simulink library "motohawk_control_primitives_lib"  (Simulink 7.5)
settings: Solver=ode45  SolverMode=SingleTasking  StartTime=0.0  StopTime=10.0  RelTol=1e-3
undefined symbols (not defined in the file): group, motohawk_vardec_config_group, motohawk_vardec_path, p, samp_time, SampleTime
libraries: MotoHawk_lib x103, motohawk_control_primitives_lib x29, simulink x11, AutoDoc_lib x4
(part 2 of 4)

== system motohawk_control_primitives_lib/Handoff Alpha ==
  note: Prevent divide by zero
  note: Convert a boolean input signal
      | to a more slowly ramping 'alpha' from 0 to 1
  in : Inport  OutDataType=sfix(16)  OutScaling=2^0
  up_tau : Inport  Port=2  OutDataType=sfix(16)  OutScaling=2^0
  down_tau : Inport  Port=3  OutDataType=sfix(16)  OutScaling=2^0
  Constant : Constant  Value=0  OutDataType=sfix(16)  OutScaling=2^0  OutDataTypeStr=Inherit: Inherit via back propagation
  Constant1 : Constant  OutDataType=sfix(16)  OutScaling=2^0  OutDataTypeStr=Inherit: Inherit via back propagation
  Multiport Switch : MultiPortSwitch  DataPortOrder=Zero-based contiguous  Inputs=2  zeroidx=on  SaturateOnIntegerOverflow=on  InputSameDT=on
  Product : Product  Inputs=*/  OutDataType=sfix(16)  OutScaling=2^0  SaturateOnIntegerOverflow=on  InputSameDT=on  OutDataTypeStr=Inherit: Same as first input
  Product1 : Product  Inputs=*/  OutDataType=sfix(16)  OutScaling=2^0  SaturateOnIntegerOverflow=on  InputSameDT=on  OutDataTypeStr=Inherit: Same as first input
  Ramp Down : Gain  Gain=-1  ParameterDataType=sfix(16)  ParameterScaling=2^0  OutDataType=sfix(16)  OutScaling=2^0  SaturateOnIntegerOverflow=on  OutDataTypeStr=Inherit: Same as input  ParamDataTypeStr=Inherit: Same as input
  Saturation : motohawk_control_primitives_lib/Saturation
  Signal Specification : SignalSpecification  DataType=boolean  OutDataType=sfix(16)  OutScaling=2^0  OutDataTypeStr=boolean
  Sum : Sum  Inputs=|++  OutDataType=sfix(16)  OutScaling=2^0  SaturateOnIntegerOverflow=on  InputSameDT=on
  Switch : Switch  Criteria=u2 > Threshold  SaturateOnIntegerOverflow=on  InputSameDT=on
  Switch1 : Switch  Criteria=u2 > Threshold  SaturateOnIntegerOverflow=on  InputSameDT=on
  motohawk_delta_time : MotoHawk_lib/Extra Development Blocks/motohawk_delta_time  samp_time=samp_time  init_val=0
  state : UnitDelay  SampleTime=-1
  alpha : Outport  OutDataType=sfix(16)  OutScaling=2^0
  wires:
  up_tau/1 -> Switch1/1, Switch1/2
  Switch1/1 -> Product1/2
  down_tau/1 -> Switch/1, Switch/2
  Switch/1 -> Product/2
  Signal Specification/1 -> Multiport Switch/1
  Ramp Down/1 -> Multiport Switch/2
  Saturation/1 -> alpha/1, state/1
  Constant1/1 -> Saturation/3
  Constant/1 -> Saturation/2
  state/1 -> Sum/2
  Sum/1 -> Saturation/1
  Multiport Switch/1 -> Sum/1
  Product1/1 -> Multiport Switch/3
  Product/1 -> Ramp Down/1
  in/1 -> Signal Specification/1
  motohawk_delta_time/1 -> Switch1/3, Product1/1, Switch/3, Product/1

== system motohawk_control_primitives_lib/Hysterisis ==
  HiThresh : Inport  OutDataType=sfix(16)  OutScaling=2^0
  LowThresh : Inport  Port=2  OutDataType=sfix(16)  OutScaling=2^0
  Signal : Inport  Port=3  OutDataType=sfix(16)  OutScaling=2^0
  Hysteresis : Subsystem
  LT : RelationalOperator  ZeroCross=off  InputSameDT=on
  LT1 : RelationalOperator  Operator=<=  ZeroCross=off  InputSameDT=on
  Logical Operator : Logic  Operator=NOT
  Switch2 : Switch  Threshold=1  ZeroCross=off  InputSameDT=on
  Threshold : Outport  OutDataType=sfix(16)  OutScaling=2^0
  wires:
  LT/1 -> Hysteresis/1(Hi)  "AboveHiTarget"
  LT1/1 -> Hysteresis/2(Lo)  "BelowLoTarget"
  Hysteresis/1("Out (Lo=0, Hi=1)") -> Logical Operator/1
  Logical Operator/1 -> Switch2/2
  HiThresh/1 -> Switch2/1, LT/2
  Switch2/1 -> Threshold/1
  LowThresh/1 -> Switch2/3, LT1/2
  Signal/1 -> LT/1, LT1/1

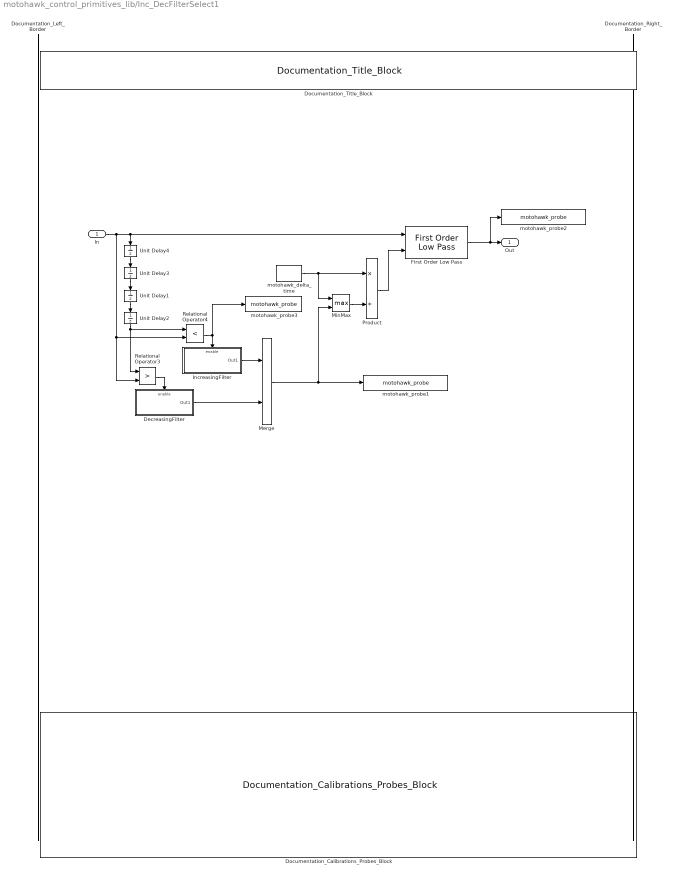
== system motohawk_control_primitives_lib/Inc_DecFilterSelect1 ==
  In : Inport  OutDataType=sfix(16)  OutScaling=2^0
  DecreasingFilter : Subsystem  TreatAsAtomicUnit=on
  Documentation_Calibrations_Probes_Block : AutoDoc_lib/Documentation_Calibrations_Probes_Block
  Documentation_Left_Border : AutoDoc_lib/Documentation_Left_Border  layout=Portrait
  Documentation_Right_Border : AutoDoc_lib/Documentation_Right_Border  layout=Portrait
  Documentation_Title_Block : AutoDoc_lib/Documentation_Title_Block
  First Order Low Pass : motohawk_control_primitives_lib/First Order Low Pass
  IncreasingFilter : Subsystem  TreatAsAtomicUnit=on
  Merge : Merge
  MinMax : MinMax  Function=max  Inputs=2  OutDataType=sfix(16)  OutScaling=2^0  SaturateOnIntegerOverflow=on  InputSameDT=on
  Product : Product  Inputs=*/  OutDataType=sfix(16)  OutScaling=2^0  SaturateOnIntegerOverflow=on  InputSameDT=on  OutDataTypeStr=Inherit: Same as first input
  Relational Operator3 : RelationalOperator  Operator=>  LogicOutDataTypeMode=boolean  OutDataTypeStr=boolean
  Relational Operator4 : RelationalOperator  Operator=<  LogicOutDataTypeMode=boolean  OutDataTypeStr=boolean
  Unit Delay{1..4} (4 alike) : UnitDelay  SampleTime=-1
  motohawk_delta_time : MotoHawk_lib/Extra Development Blocks/motohawk_delta_time  samp_time=.005  init_val=.005
  motohawk_probe1 : MotoHawk_lib/Calibration & Probing Blocks/motohawk_probe  nam=[nam 'FilterConst']  show_more=on  name_source=Use Parameter  read_level=1  view_as=Number  enum_struct={'Disabled', 'Enabled'}  vector_style=Wide Row  use_help_units=off  help=''  units=''  use_header_enum=off  row_header_enum={}  col_header_enum={}  use_precision=off  precision=''  gain=1  offset=0  exp=1  use_mototune_group=on  mototune_group=grp_dis
  motohawk_probe2 : MotoHawk_lib/Calibration & Probing Blocks/motohawk_probe  nam=[nam 'Filtered']  show_more=on  name_source=Use Parameter  read_level=1  view_as=Number  enum_struct={'Disabled', 'Enabled'}  vector_style=Wide Row  use_help_units=off  help=''  units=''  use_header_enum=off  row_header_enum={}  col_header_enum={}  use_precision=off  precision=''  gain=1  offset=0  exp=1  use_mototune_group=on  mototune_group=grp_dis
  motohawk_probe3 : MotoHawk_lib/Calibration & Probing Blocks/motohawk_probe  nam=[nam 'Direction']  show_more=on  name_source=Use Parameter  read_level=1  view_as=Enumeration  enum_struct={'Decreasing', 'Increasing'}  vector_style=Wide Row  use_help_units=on  help=''  units=''  use_header_enum=off  row_header_enum={}  col_header_enum={}  use_precision=off  precision=''  gain=1  offset=0  exp=1  use_mototune_group=on  mototune_group=grp_dis
  Out : Outport  OutDataType=sfix(16)  OutScaling=2^0
  wires:
  Unit Delay4/1 -> Unit Delay3/1
  Unit Delay3/1 -> Unit Delay1/1
  Unit Delay1/1 -> Unit Delay2/1
  Unit Delay2/1 -> Relational Operator4/1, Relational Operator3/1
  Product/1 -> First Order Low Pass/2
  First Order Low Pass/1 -> Out/1, motohawk_probe2/1
  motohawk_delta_time/1 -> MinMax/1, Product/1
  MinMax/1 -> Product/2
  Merge/1 -> MinMax/2, motohawk_probe1/1
  Relational Operator4/1 -> motohawk_probe3/1, IncreasingFilter/Enable
  Relational Operator3/1 -> DecreasingFilter/Enable
  DecreasingFilter/1(Out1) -> Merge/2
  IncreasingFilter/1(Out1) -> Merge/1
  In/1 -> First Order Low Pass/1, Unit Delay4/1, Relational Operator3/2, Relational Operator4/2

== system motohawk_control_primitives_lib/Integrator ==
  note: Discrete Integrator,
      | with output and state saturation.
  In : Inport  OutDataType=sfix(16)  OutScaling=2^0
  Rst : Inport  Port=2  OutDataType=sfix(16)  OutScaling=2^0
  IC : Inport  Port=3  OutDataType=sfix(16)  OutScaling=2^0
  Min : Inport  Port=4  OutDataType=sfix(16)  OutScaling=2^0
  Max : Inport  Port=5  OutDataType=sfix(16)  OutScaling=2^0
  Data Type Conversion : DataTypeConversion  OutDataTypeMode=boolean  OutDataType=sfix(16)  OutScaling=2^0  OutDataTypeStr=boolean  RndMeth=Zero
  Product : Product  OutDataType=sfix(16)  OutScaling=2^0  SaturateOnIntegerOverflow=on  InputSameDT=on  OutDataTypeStr=Inherit: Same as first input
  Saturation : motohawk_control_primitives_lib/Saturation
  Sum : Sum  Inputs=++|  OutDataType=sfix(16)  OutScaling=2^0  SaturateOnIntegerOverflow=on  InputSameDT=on
  Switch1 : Switch  Threshold=1  ZeroCross=off  SaturateOnIntegerOverflow=on  InputSameDT=on
  Unit Delay : UnitDelay  SampleTime=-1
  motohawk_delta_time : MotoHawk_lib/Extra Development Blocks/motohawk_delta_time  samp_time=-1  init_val=0
  Out : Outport  OutDataType=sfix(16)  OutScaling=2^0
  wires:
  Saturation/1 -> Unit Delay/1
  Sum/1 -> Saturation/1
  Switch1/1 -> Out/1, Sum/1
  motohawk_delta_time/1 -> Product/2
  In/1 -> Product/1
  Product/1 -> Sum/2
  Unit Delay/1 -> Switch1/3
  Rst/1 -> Data Type Conversion/1
  Data Type Conversion/1 -> Switch1/2
  Min/1 -> Saturation/2
  Max/1 -> Saturation/3
  IC/1 -> Switch1/1

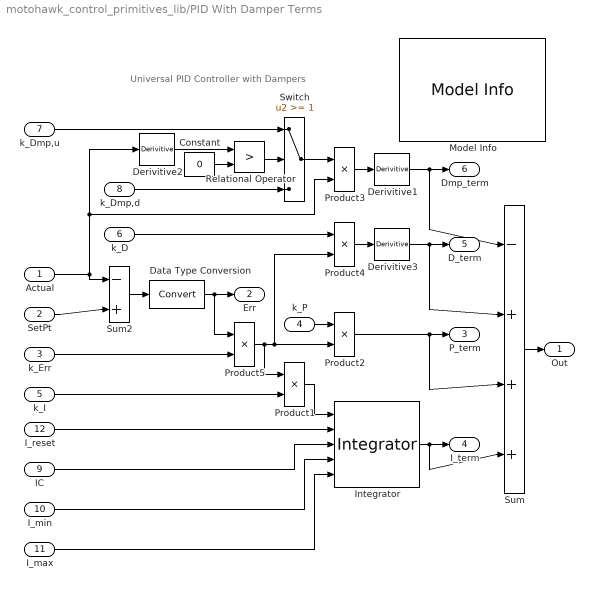
== system motohawk_control_primitives_lib/PID With Damper Terms ==
  note: Universal PID Controller
      | with Dampers
  Actual : Inport  OutDataType=sfix(16)  OutScaling=2^0
  SetPt : Inport  Port=2  OutDataType=sfix(16)  OutScaling=2^0
  k_Err : Inport  Port=3  OutDataType=sfix(16)  OutScaling=2^0
  k_P : Inport  Port=4  OutDataType=sfix(16)  OutScaling=2^0
  k_I : Inport  Port=5  OutDataType=sfix(16)  OutScaling=2^0
  k_D : Inport  Port=6  OutDataType=sfix(16)  OutScaling=2^0
  k_Dmp,u : Inport  Port=7  OutDataType=sfix(16)  OutScaling=2^0
  k_Dmp,d : Inport  Port=8  OutDataType=sfix(16)  OutScaling=2^0
  IC : Inport  Port=9  OutDataType=sfix(16)  OutScaling=2^0
  I_min : Inport  Port=10  OutDataType=sfix(16)  OutScaling=2^0
  I_max : Inport  Port=11  OutDataType=sfix(16)  OutScaling=2^0
  I_reset : Inport  Port=12  OutDataType=sfix(16)  OutScaling=2^0
  Constant : Constant  Value=0  OutDataType=sfix(16)  OutScaling=2^0  OutDataTypeStr=Inherit: Inherit via back propagation
  Data Type Conversion : DataTypeConversion  OutDataType=sfix(16)  OutScaling=2^0  SaturateOnIntegerOverflow=on  RndMeth=Zero
  Derivitive1 : motohawk_control_primitives_lib/Derivitive  samp_time=samp_time
  Derivitive2 : motohawk_control_primitives_lib/Derivitive  samp_time=samp_time
  Derivitive3 : motohawk_control_primitives_lib/Derivitive  samp_time=samp_time
  Integrator : motohawk_control_primitives_lib/Integrator  samp_time=samp_time
  Model Info : simulink/Model-Wide Utilities/Model Info  InitialBlockCM=None  BlockCM=None  Frame=on  DisplayStringWithTags=|  HorizontalTextAlignment=Center  LeftAlignmentValue=0.5  SourceBlockDiagram=motohawk_control_primitives_lib  TagMaxNumber=20
      | Model Info:
      | Author: Suhre, Poorman
      | %<Created>
      | %<ModifiedDate>
      | Version: %<ModelVersion>
      | MotoTron Confidential
      | and Propietary
  Product{1..5} (5 alike) : Product  OutDataType=sfix(16)  OutScaling=2^0  InputSameDT=on  OutDataTypeStr=Inherit: Same as first input
  Relational Operator : RelationalOperator  Operator=>  ZeroCross=off  InputSameDT=on
  Sum : Sum  Inputs=-|+|+|+  OutDataType=sfix(16)  OutScaling=2^0  SaturateOnIntegerOverflow=on  InputSameDT=on  OutDataTypeStr=Inherit: Same as first input
  Sum2 : Sum  Inputs=-|+  OutDataType=sfix(16)  OutScaling=2^0  SaturateOnIntegerOverflow=on  InputSameDT=on  OutDataTypeStr=Inherit: Same as first input
  Switch : Switch  Threshold=1  ZeroCross=off  InputSameDT=on
  Out : Outport  OutDataType=sfix(16)  OutScaling=2^0
  Err : Outport  Port=2  OutDataType=sfix(16)  OutScaling=2^0
  P_term : Outport  Port=3  OutDataType=sfix(16)  OutScaling=2^0
  I_term : Outport  Port=4  OutDataType=sfix(16)  OutScaling=2^0
  D_term : Outport  Port=5  OutDataType=sfix(16)  OutScaling=2^0
  Dmp_term : Outport  Port=6  OutDataType=sfix(16)  OutScaling=2^0
  wires:
  Product3/1 -> Derivitive1/1
  k_Dmp,u/1 -> Switch/1
  k_Dmp,d/1 -> Switch/3
  Switch/1 -> Product3/1
  Derivitive2/1 -> Relational Operator/1
  Relational Operator/1 -> Switch/2
  Constant/1 -> Relational Operator/2
  I_max/1 -> Integrator/5
  I_min/1 -> Integrator/4
  Data Type Conversion/1 -> Product5/1, Err/1
  k_Err/1 -> Product5/2
  I_reset/1 -> Integrator/2
  Actual/1 -> Sum2/1, Derivitive2/1, Product3/2
  k_P/1 -> Product2/1
  k_I/1 -> Product1/2
  Product1/1 -> Integrator/1
  Product2/1 -> P_term/1, Sum/3
  Integrator/1 -> I_term/1, Sum/4
  Sum/1 -> Out/1
  IC/1 -> Integrator/3
  Product5/1 -> Product1/1, Product2/2, Product4/2
  Sum2/1 -> Data Type Conversion/1
  SetPt/1 -> Sum2/2
  k_D/1 -> Product4/1
  Product4/1 -> Derivitive3/1
  Derivitive3/1 -> D_term/1, Sum/2
  Derivitive1/1 -> Dmp_term/1, Sum/1

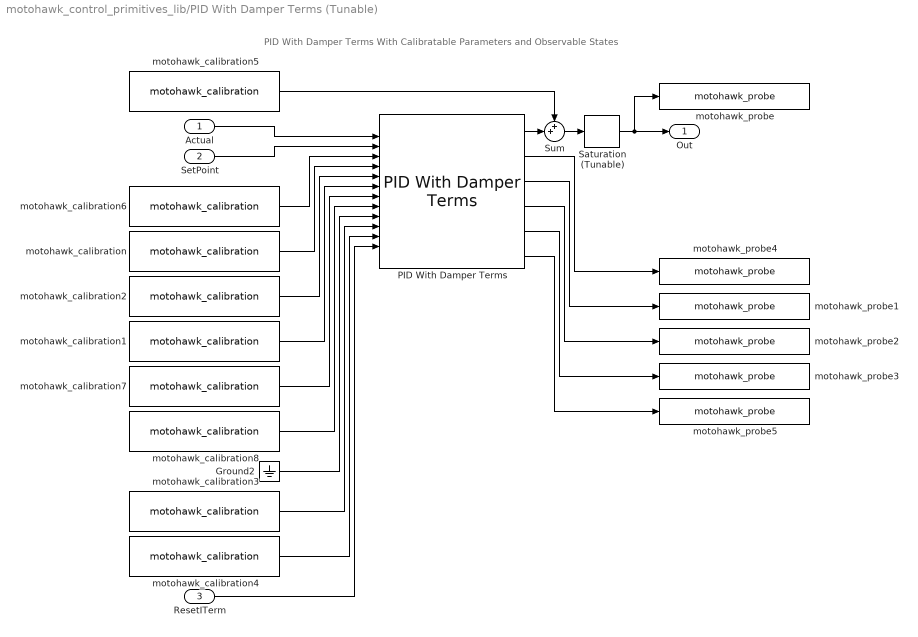
== system motohawk_control_primitives_lib/PID With Damper Terms (Tunable) ==
  note: PID With Damper Terms
      | With Calibratable Parameters and Observable States
  Actual : Inport  OutDataType=sfix(16)  OutScaling=2^0
  SetPoint : Inport  Port=2  OutDataType=sfix(16)  OutScaling=2^0
  ResetITerm : Inport  Port=3  OutDataType=sfix(16)  OutScaling=2^0
  Ground2 : Ground
  PID With Damper Terms : motohawk_control_primitives_lib/PID With Damper Terms  Description=|  samp_time=SampleTime
      | /* Name: ErrorGain Unit:mult ClassID:VAR StorageID:FLASH Access:RW4+RW3+NA2+NA1 TypeID:UINT4                   
      |    Gain:0.000000001 Min:0.000000000 Max:4.000000000 Format:10.9 UpdateID:REMOTE Help:"This gain is applied to "
      |    "the error term before it is used to calculate the P, I and D terms." VardecSig:6C */                       
      |                                                                                                                
      | /* Name: ITermLowerLim Unit:0 ClassID:VAR StorageID:FLASH Access:RW4+RW3+NA2+NA1 TypeID:SINT2 Gain:0.1         
      |    Min:-3276.8 Max:3276.7 Format:5.1 UpdateID:REMOTE Help:"Lower limit on the I-term value." VardecSig:6C */   
      |                                                                                                                
      | /* Name: ITermUpperLim ClassID:VAR StorageID:FLASH Access:RW4+RW3+NA2+NA1 TypeID:SINT2 Gain:0.1 Min:-3276.8    
      |    Max:3276.7 Format:5.1 UpdateID:REMOTE Help:"Upper limit on I-term value." VardecSig:6C */                   
      |                                                                                                                
      | /* Name: PIDOutLowerLim ClassID:VAR StorageID:FLASH Access:RW4+RW3+NA2+NA1 TypeID:SINT2 Gain:0.1               
      |    Min:-3276.8 Max:3276.7 Format:5.1 UpdateID:REMOTE Help:"Lower limit on PID output." VardecSig:6C */         
      |                                                                                                                
      | /* Name: PIDOutUpperLim ClassID:VAR StorageID:FLASH Access:RW4+RW3+NA2+NA1 TypeID:SINT2 Gain:0.1               
      |    Min:-3276.8 Max:3276.7 Format:3.1 UpdateID:REMOTE Help:"Upper limit on PID output." VardecSig:6C */         
      |                                                                                                                
      | /* Name: PIDError ClassID:VAR StorageID:RAM Access:RO4+RO3+NA2+NA1 TypeID:SINT2 Gain:1 Min:-32768.00           
      |    Max:32767.00 Format:4.2 UpdateID:BACKGND Help:"Current controller error input value." VardecSig:6C */       
      |                                                                                                                
      | /* Name: PTerm ClassID:VAR StorageID:RAM Access:RO4+RO3+NA2+NA1 TypeID:SINT2 Gain:1 Min:-32768.00              
      |    Max:32767.00 Format:4.2 UpdateID:BACKGND Help:"Current P-term value" VardecSig:6C */                        
      |                                                                                                                
      | /* Name: ITerm ClassID:VAR StorageID:RAM Access:RO4+RO3+NA2+NA1 TypeID:SINT2 Gain:1 Min:-32768.00              
      |    Max:32767.00 Format:4.2 UpdateID:BACKGND Help:"Current I-term value" VardecSig:6C */                        
      |                                                                                                                
      | /* Name: DTerm ClassID:VAR StorageID:RAM Access:RO4+RO3+NA2+NA1 TypeID:SINT2 Gain:1 Min:-32768.00              
      |    Max:32767.00 Format:4.2 UpdateID:BACKGND Help:"Current D-term value" VardecSig:6C */                        
      |                                                                                                                
      | /* Name: DamperTerm ClassID:VAR StorageID:RAM Access:RO4+RO3+NA2+NA1 TypeID:SINT2 Gain:1 Min:-32768.00         
      |    Max:32767.00 Format:4.2 UpdateID:BACKGND Help:"Current Damper-term value" VardecSig:6C */                   
      |                                                                                                                
      | /* Name: PIDOutput ClassID:VAR StorageID:FLASH Access:RW4+RW3+NA2+NA1 TypeID:SINT2 Gain:1 Min:-32768.00        
      |    Max:32767.00 Format:4.2 UpdateID:REMOTE Help:"PID current output." VardecSig:6C */
  Saturation (Tunable) : motohawk_control_primitives_lib/Saturation (Tunable)  prefix=prefix  units=units  grp=grp
  Sum : Sum  Inputs=++|  OutDataType=sfix(16)  OutScaling=2^0  InputSameDT=on
  motohawk_calibration : MotoHawk_lib/Calibration & Probing Blocks/motohawk_calibration  nam=[prefix 'PGain']  val=1  storage=Calibration  show_more=on  name_source=Use Parameter  data_type=Inherit from 'Default Value'  read_level=1  write_level=1  ovr_cals=on  view_as=Number  enum_struct={'Disabled', 'Enabled'}  vector_style=Wide Row  use_help_units=on  help='PID Proportional Gain'  units='mult'  use_header_enum=off  row_header_enum={}  col_header_enum={}  use_min_max=off  min_val=-inf  max_val=inf  use_precision=off  precision=''  gain=1  offset=0  exp=1  use_mototune_group=on  mototune_group=grp
  motohawk_calibration1 : MotoHawk_lib/Calibration & Probing Blocks/motohawk_calibration  nam=[prefix 'DGain']  val=1  storage=Calibration  show_more=on  name_source=Use Parameter  data_type=Inherit from 'Default Value'  read_level=1  write_level=1  ovr_cals=on  view_as=Number  enum_struct={'Disabled', 'Enabled'}  vector_style=Wide Row  use_help_units=on  help='PID Derivative Gain'  units='mult'  use_header_enum=off  row_header_enum={}  col_header_enum={}  use_min_max=off  min_val=-inf  max_val=inf  use_precision=off  precision=''  gain=1  offset=0  exp=1  use_mototune_group=on  mototune_group=grp
  motohawk_calibration2 : MotoHawk_lib/Calibration & Probing Blocks/motohawk_calibration  nam=[prefix 'IGain']  val=1  storage=Calibration  show_more=on  name_source=Use Parameter  data_type=Inherit from 'Default Value'  read_level=1  write_level=1  ovr_cals=on  view_as=Number  enum_struct={'Disabled', 'Enabled'}  vector_style=Wide Row  use_help_units=on  help='PID Integral Gain'  units='mult'  use_header_enum=off  row_header_enum={}  col_header_enum={}  use_min_max=off  min_val=-inf  max_val=inf  use_precision=off  precision=''  gain=1  offset=0  exp=1  use_mototune_group=on  mototune_group=grp
  motohawk_calibration3 : MotoHawk_lib/Calibration & Probing Blocks/motohawk_calibration  nam=[prefix 'IMin']  val=0  storage=Calibration  show_more=on  name_source=Use Parameter  data_type=Inherit from 'Default Value'  read_level=1  write_level=1  ovr_cals=on  view_as=Number  enum_struct={'Disabled', 'Enabled'}  vector_style=Wide Row  use_help_units=on  help='PID Integrator Lower Limit'  units=units  use_header_enum=off  row_header_enum={}  col_header_enum={}  use_min_max=off  min_val=-inf  max_val=inf  use_precision=off  precision=''  gain=1  offset=0  exp=1  use_mototune_group=on  mototune_group=grp
  motohawk_calibration4 : MotoHawk_lib/Calibration & Probing Blocks/motohawk_calibration  nam=[prefix 'IMax']  val=1  storage=Calibration  show_more=on  name_source=Use Parameter  data_type=Inherit from 'Default Value'  read_level=1  write_level=1  ovr_cals=on  view_as=Number  enum_struct={'Disabled', 'Enabled'}  vector_style=Wide Row  use_help_units=on  help='PID Integrator Upper Limit'  units=units  use_header_enum=off  row_header_enum={}  col_header_enum={}  use_min_max=off  min_val=-inf  max_val=inf  use_precision=off  precision=''  gain=1  offset=0  exp=1  use_mototune_group=on  mototune_group=grp
  motohawk_calibration5 : MotoHawk_lib/Calibration & Probing Blocks/motohawk_calibration  nam=[prefix 'DCOffset']  val=0  storage=Calibration  show_more=on  name_source=Use Parameter  data_type=Inherit from 'Default Value'  read_level=1  write_level=1  ovr_cals=on  view_as=Number  enum_struct={'Disabled', 'Enabled'}  vector_style=Wide Row  use_help_units=on  help='PID Output DC Offset'  units=units  use_header_enum=off  row_header_enum={}  col_header_enum={}  use_min_max=off  min_val=-inf  max_val=inf  use_precision=off  precision=''  gain=1  offset=0  exp=1  use_mototune_group=on  mototune_group=grp
  motohawk_calibration6 : MotoHawk_lib/Calibration & Probing Blocks/motohawk_calibration  nam=[prefix 'ErrorGain']  val=1  storage=Calibration  show_more=on  name_source=Use Parameter  data_type=Inherit from 'Default Value'  read_level=1  write_level=1  ovr_cals=on  view_as=Number  enum_struct={'Disabled', 'Enabled'}  vector_style=Wide Row  use_help_units=on  help='PID Error Gain'  units='mult'  use_header_enum=off  row_header_enum={}  col_header_enum={}  use_min_max=off  min_val=-inf  max_val=inf  use_precision=off  precision=''  gain=1  offset=0  exp=1  use_mototune_group=on  mototune_group=grp
  motohawk_calibration7 : MotoHawk_lib/Calibration & Probing Blocks/motohawk_calibration  nam=[prefix 'DampGainUp']  val=1  storage=Calibration  show_more=on  name_source=Use Parameter  data_type=Inherit from 'Default Value'  read_level=1  write_level=1  ovr_cals=on  view_as=Number  enum_struct={'Disabled', 'Enabled'}  vector_style=Wide Row  use_help_units=on  help='PID Damper Gain - Up Direction'  units='mult'  use_header_enum=off  row_header_enum={}  col_header_enum={}  use_min_max=off  min_val=-inf  max_val=inf  use_precision=off  precision=''  gain=1  offset=0  exp=1  use_mototune_group=on  mototune_group=grp
  motohawk_calibration8 : MotoHawk_lib/Calibration & Probing Blocks/motohawk_calibration  nam=[prefix 'DampGainDown']  val=1  storage=Calibration  show_more=on  name_source=Use Parameter  data_type=Inherit from 'Default Value'  read_level=1  write_level=1  ovr_cals=on  view_as=Number  enum_struct={'Disabled', 'Enabled'}  vector_style=Wide Row  use_help_units=on  help='PID Damper Gain - Down Direction'  units='mult'  use_header_enum=off  row_header_enum={}  col_header_enum={}  use_min_max=off  min_val=-inf  max_val=inf  use_precision=off  precision=''  gain=1  offset=0  exp=1  use_mototune_group=on  mototune_group=grp
  motohawk_probe : MotoHawk_lib/Calibration & Probing Blocks/motohawk_probe  nam=[prefix 'Out']  show_more=on  name_source=Use Parameter  read_level=1  view_as=Number  enum_struct={'Disabled', 'Enabled'}  vector_style=Wide Row  use_help_units=on  help='PID Final Output'  units=units  use_header_enum=off  row_header_enum={}  col_header_enum={}  use_precision=off  precision=''  gain=1  offset=0  exp=1  use_mototune_group=on  mototune_group=grp
  motohawk_probe1 : MotoHawk_lib/Calibration & Probing Blocks/motohawk_probe  nam=[prefix 'PTerm']  show_more=on  name_source=Use Parameter  read_level=1  view_as=Number  enum_struct={'Disabled', 'Enabled'}  vector_style=Wide Row  use_help_units=on  help='PID Proportional Term'  units=units  use_header_enum=off  row_header_enum={}  col_header_enum={}  use_precision=off  precision=''  gain=1  offset=0  exp=1  use_mototune_group=on  mototune_group=grp
  motohawk_probe2 : MotoHawk_lib/Calibration & Probing Blocks/motohawk_probe  nam=[prefix 'ITerm']  show_more=on  name_source=Use Parameter  read_level=1  view_as=Number  enum_struct={'Disabled', 'Enabled'}  vector_style=Wide Row  use_help_units=on  help='PID Integrator Term'  units=units  use_header_enum=off  row_header_enum={}  col_header_enum={}  use_precision=off  precision=''  gain=1  offset=0  exp=1  use_mototune_group=on  mototune_group=grp
  motohawk_probe3 : MotoHawk_lib/Calibration & Probing Blocks/motohawk_probe  nam=[prefix 'DTerm']  show_more=on  name_source=Use Parameter  read_level=1  view_as=Number  enum_struct={'Disabled', 'Enabled'}  vector_style=Wide Row  use_help_units=on  help='PID Derivative Term'  units=units  use_header_enum=off  row_header_enum={}  col_header_enum={}  use_precision=off  precision=''  gain=1  offset=0  exp=1  use_mototune_group=on  mototune_group=grp
  motohawk_probe4 : MotoHawk_lib/Calibration & Probing Blocks/motohawk_probe  nam=[prefix 'Error']  show_more=on  name_source=Use Parameter  read_level=1  view_as=Number  enum_struct={'Disabled', 'Enabled'}  vector_style=Wide Row  use_help_units=on  help='PID Error Term'  units=units  use_header_enum=off  row_header_enum={}  col_header_enum={}  use_precision=off  precision=''  gain=1  offset=0  exp=1  use_mototune_group=on  mototune_group=grp
  motohawk_probe5 : MotoHawk_lib/Calibration & Probing Blocks/motohawk_probe  nam=[prefix 'DampTerm']  show_more=on  name_source=Use Parameter  read_level=1  view_as=Number  enum_struct={'Disabled', 'Enabled'}  vector_style=Wide Row  use_help_units=on  help='PID Damper Term'  units=units  use_header_enum=off  row_header_enum={}  col_header_enum={}  use_precision=off  precision=''  gain=1  offset=0  exp=1  use_mototune_group=on  mototune_group=grp
  Out : Outport  OutDataType=sfix(16)  OutScaling=2^0
  wires:
  motohawk_calibration5/1 -> Sum/1
  Sum/1 -> Saturation (Tunable)/1
  ResetITerm/1 -> PID With Damper Terms/12
  Ground2/1 -> PID With Damper Terms/9
  motohawk_calibration1/1 -> PID With Damper Terms/6
  motohawk_calibration2/1 -> PID With Damper Terms/5
  motohawk_calibration/1 -> PID With Damper Terms/4
  PID With Damper Terms/3 -> motohawk_probe1/1
  Actual/1 -> PID With Damper Terms/1
  SetPoint/1 -> PID With Damper Terms/2
  PID With Damper Terms/1 -> Sum/2
  motohawk_calibration6/1 -> PID With Damper Terms/3
  motohawk_calibration3/1 -> PID With Damper Terms/10
  motohawk_calibration4/1 -> PID With Damper Terms/11
  PID With Damper Terms/4 -> motohawk_probe2/1
  PID With Damper Terms/5 -> motohawk_probe3/1
  PID With Damper Terms/2 -> motohawk_probe4/1
  motohawk_calibration7/1 -> PID With Damper Terms/7
  motohawk_calibration8/1 -> PID With Damper Terms/8
  PID With Damper Terms/6 -> motohawk_probe5/1
  Saturation (Tunable)/1 -> Out/1, motohawk_probe/1

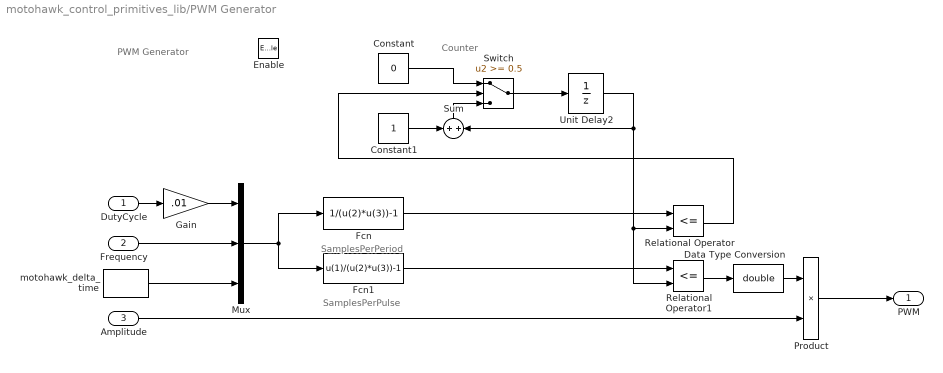
== system motohawk_control_primitives_lib/PWM Generator ==
  note: Counter
  note: PWM Generator
  note: SamplesPerPulse
  note: SamplesPerPeriod
  DutyCycle : Inport  OutDataType=sfix(16)  OutScaling=2^0
  Frequency : Inport  Port=2  OutDataType=sfix(16)  OutScaling=2^0
  Amplitude : Inport  Port=3  OutDataType=sfix(16)  OutScaling=2^0
  Enable : EnablePort  StatesWhenEnabling=reset
  Constant : Constant  Value=0  OutDataType=sfix(16)  OutScaling=2^0
  Constant1 : Constant  OutDataType=sfix(16)  OutScaling=2^0
  Data Type Conversion : DataTypeConversion  OutDataTypeMode=double  OutDataType=sfix(16)  OutScaling=2^0  OutDataTypeStr=double  SaturateOnIntegerOverflow=on  RndMeth=Zero
  Fcn : Fcn  Expr=1/(u(2)*u(3))-1
  Fcn1 : Fcn  Expr=u(1)/(u(2)*u(3))-1
  Gain : Gain  Gain=.01  ParameterDataType=sfix(16)  ParameterScaling=2^0  OutDataType=sfix(16)  OutScaling=2^0  SaturateOnIntegerOverflow=on  OutDataTypeStr=Inherit: Same as input  ParamDataTypeStr=Inherit: Same as input
  Mux : Mux  Inputs=3
  Product : Product  OutDataType=sfix(16)  OutScaling=2^0  SaturateOnIntegerOverflow=on  OutDataTypeStr=Inherit: Same as first input
  Relational Operator : RelationalOperator  Operator=<=
  Relational Operator1 : RelationalOperator  Operator=<=
  Sum : Sum  OutDataType=sfix(16)  OutScaling=2^0  SaturateOnIntegerOverflow=on  InputSameDT=on  OutDataTypeStr=Inherit: Same as first input
  Switch : Switch  Threshold=0.5  SaturateOnIntegerOverflow=on  InputSameDT=on
  Unit Delay2 : UnitDelay  SampleTime=-1
  motohawk_delta_time : MotoHawk_lib/Extra Development Blocks/motohawk_delta_time  samp_time=-1  init_val=.005
  PWM : Outport  OutDataType=sfix(16)  OutScaling=2^0  OutputWhenDisabled=reset  InitialOutput=0
  wires:
  Relational Operator/1 -> Switch/2
  Constant1/1 -> Sum/1
  Gain/1 -> Mux/1
  Data Type Conversion/1 -> Product/1
  Unit Delay2/1 -> Relational Operator1/2, Relational Operator/2, Sum/2
  Switch/1 -> Unit Delay2/1
  Constant/1 -> Switch/1
  Sum/1 -> Switch/3
  Amplitude/1 -> Product/2
  Product/1 -> PWM/1
  Relational Operator1/1 -> Data Type Conversion/1
  Fcn1/1 -> Relational Operator1/1
  Fcn/1 -> Relational Operator/1
  Mux/1 -> Fcn1/1, Fcn/1
  motohawk_delta_time/1 -> Mux/3
  Frequency/1 -> Mux/2
  DutyCycle/1 -> Gain/1

== system motohawk_control_primitives_lib/Per Cylinder Tables ==
  y_Idx : Inport  OutDataType=sfix(16)  OutScaling=2^0
  X_Idx : Inport  Port=2  OutDataType=sfix(16)  OutScaling=2^0
  Cyl : Inport  Port=3  OutDataType=sfix(16)  OutScaling=2^0
  Cyl1 : Subsystem  TreatAsAtomicUnit=on
  Cyl2 : Subsystem  TreatAsAtomicUnit=on
  Cyl3 : Subsystem  TreatAsAtomicUnit=on
  Cyl4 : Subsystem  TreatAsAtomicUnit=on
  Cyl5 : Subsystem  TreatAsAtomicUnit=on
  Cyl6 : Subsystem  TreatAsAtomicUnit=on
  Data Type Conversion : DataTypeConversion  OutDataTypeMode=uint8  OutDataType=sfix(16)  OutScaling=2^0  OutDataTypeStr=uint8  SaturateOnIntegerOverflow=on  RndMeth=Zero
  Multiport Switch : MultiPortSwitch  Inputs=6  zeroidx=off  SaturateOnIntegerOverflow=on
  Switch Case : SwitchCase  CaseConditions={1,2,3,4,5,6}  ShowDefaultCase=off
  Out1 : Outport  OutDataType=sfix(16)  OutScaling=2^0
  wires:
  Multiport Switch/1 -> Out1/1
  Cyl6/1(Value) -> Multiport Switch/7
  Cyl5/1(Value) -> Multiport Switch/6
  Cyl4/1(Value) -> Multiport Switch/5
  Cyl3/1(Value) -> Multiport Switch/4
  Cyl2/1(Value) -> Multiport Switch/3
  Cyl1/1(Value) -> Multiport Switch/2
  Data Type Conversion/1 -> Multiport Switch/1, Switch Case/1
  Switch Case/6 -> Cyl6/Action
  Switch Case/5 -> Cyl5/Action
  Switch Case/4 -> Cyl4/Action
  Switch Case/3 -> Cyl3/Action
  Switch Case/2 -> Cyl2/Action
  Switch Case/1 -> Cyl1/Action
  y_Idx/1 -> Cyl6/1(Row), Cyl5/1(Row), Cyl4/1(Row), Cyl3/1(Row), Cyl2/1(Row), Cyl1/1(Row)
  X_Idx/1 -> Cyl6/2(Col), Cyl5/2(Col), Cyl4/2(Col), Cyl3/2(Col), Cyl2/2(Col), Cyl1/2(Col)
  Cyl/1 -> Data Type Conversion/1

== system motohawk_control_primitives_lib/Polynomial (Tunable) ==
  note: Evaluate polynomial using Horner's Rule.
      |      y = polyval( p, u, [], mu )
      | where
      |      p = polynomial coefficients and
      |      mu(1) = mean and
      |      mu(2) = standard deviation of fitted data.
      | See MATLAB "help polyfit" for more.
      | Note:  Degree of polynomial is fixed at compile time.
      | MotoTune can change coefficients, centering/scaling values.
  note: Evaluate Polynomial using Horner's Rule.
  u : Inport  OutDataType=sfix(16)  OutScaling=2^0
  Constant : Constant  Value=[0 1]  OutDataType=sfix(16)  OutScaling=2^0
  Demux : Demux  Outputs=2
  Horner's Rule : Subsystem
  Product0 : Product  Inputs=*/  OutDataType=sfix(16)  OutScaling=2^0  SaturateOnIntegerOverflow=on  OutDataTypeStr=Inherit: Same as first input
  Signal Specification0 : SignalSpecification  Dimensions=2  OutDataType=sfix(16)  OutScaling=2^0
  Signal Specification1 : SignalSpecification  Dimensions=length(p)  OutDataType=sfix(16)  OutScaling=2^0
  Sum : Sum  Inputs=|+-  OutDataType=sfix(16)  OutScaling=2^0  OutDataTypeStr=Inherit: Inherit via back propagation  SaturateOnIntegerOverflow=on  InputSameDT=on
  motohawk_calibration1 : MotoHawk_lib/Calibration & Probing Blocks/motohawk_calibration  nam=[prefix 'Polynomial']  val=ones(1,numcoef)  storage=Calibration  show_more=on  name_source=Use Parameter  data_type=Inherit from 'Default Value'  read_level=1  write_level=1  ovr_cals=on  view_as=Number  enum_struct={'Disabled', 'Enabled'}  vector_style=Wide Row  use_help_units=on  help='[ A_n ... A_0 ]'  units=''  use_header_enum=off  row_header_enum={}  col_header_enum={}  use_min_max=on  min_val=-inf  max_val=inf  use_precision=on  precision='1.14'  gain=1  offset=0  exp=1  use_mototune_group=on  mototune_group=grp
  y : Outport  OutDataType=sfix(16)  OutScaling=2^0
  wires:
  Signal Specification0/1 -> Demux/1
  Signal Specification1/1 -> Horner's Rule/2(p)
  Horner's Rule/1(y) -> y/1
  motohawk_calibration1/1 -> Signal Specification1/1
  Product0/1 -> Horner's Rule/1(u_hat)
  Demux/2 -> Product0/2
  Constant/1 -> Signal Specification0/1
  Sum/1 -> Product0/1
  Demux/1 -> Sum/2
  u/1 -> Sum/1

== system motohawk_control_primitives_lib/Rising Edge ==
  note: Detect Rising Edge of Signal
      | using Discrete Unit Delay
  In : Inport  OutDataType=sfix(16)  OutScaling=2^0
  Data Type Conversion : DataTypeConversion  OutDataTypeMode=boolean  OutDataType=sfix(16)  OutScaling=2^0  OutDataTypeStr=boolean  SaturateOnIntegerOverflow=on  RndMeth=Zero
  Logical Operator : Logic
  Logical Operator1 : Logic  Operator=NOT
  Unit Delay : UnitDelay  SampleTime=-1
  Rise : Outport  OutDataType=sfix(16)  OutScaling=2^0
  wires:
  Data Type Conversion/1 -> Unit Delay/1, Logical Operator/1
  Logical Operator1/1 -> Logical Operator/2
  Unit Delay/1 -> Logical Operator1/1
  Logical Operator/1 -> Rise/1
  In/1 -> Data Type Conversion/1

== system motohawk_control_primitives_lib/Saturate Divide ==
  note: When the divisor is less than the numerator,
      | saturate and output one.
  note: This is useful when dividing dT by a Time Constant.
      | It also avoids a divide by zero.
  X : Inport  OutDataType=sfix(16)  OutScaling=2^0
  Inport : Inport  Port=2  OutDataType=sfix(16)  OutScaling=2^0
  If : If  NumInputs=2  IfExpression=u2 < u1
  Merge : Merge
  Normal Divide : Subsystem
  Output One : Subsystem
  " " : Outport  OutDataType=sfix(16)  OutScaling=2^0
  wires:
  X/1 -> Normal Divide/1(X), If/1
  Merge/1 -> " "/1
  Normal Divide/1(" ") -> Merge/1
  Output One/1(" ") -> Merge/2
  If/2 -> Normal Divide/Action
  If/1 -> Output One/Action
  Inport/1 -> Normal Divide/2(Inport), If/2

== system motohawk_control_primitives_lib/Saturation ==
  note: Output 'In' when between Min and Max,
      | and saturate against limits otherwise.
  in : Inport  OutDataType=sfix(16)  OutScaling=2^0
  min : Inport  Port=2  OutDataType=sfix(16)  OutScaling=2^0
  max : Inport  Port=3  OutDataType=sfix(16)  OutScaling=2^0
  MinMax : MinMax  Function=max  Inputs=2  OutDataType=sfix(16)  OutScaling=2^0  ZeroCross=off  SaturateOnIntegerOverflow=on  InputSameDT=on
  MinMax1 : MinMax  Inputs=2  OutDataType=sfix(16)  OutScaling=2^0  ZeroCross=off  SaturateOnIntegerOverflow=on  InputSameDT=on
  out : Outport  OutDataType=sfix(16)  OutScaling=2^0
  wires:
  MinMax/1 -> MinMax1/1
  in/1 -> MinMax/1
  min/1 -> MinMax/2
  max/1 -> MinMax1/2
  MinMax1/1 -> out/1

== system motohawk_control_primitives_lib/Saturation (Tunable) ==
  note: Calibratable wrapper around the Saturation block
  In : Inport  OutDataType=sfix(16)  OutScaling=2^0
  Saturation : motohawk_control_primitives_lib/Saturation
  motohawk_calibration : MotoHawk_lib/Calibration & Probing Blocks/motohawk_calibration  nam=[prefix 'LwrLim']  val=0  storage=Calibration  show_more=on  name_source=Use Parameter  data_type=Inherit via back propagation  read_level=1  write_level=1  ovr_cals=on  view_as=Number  enum_struct={'Disabled', 'Enabled'}  vector_style=Wide Row  use_help_units=off  help='Lower Limit Value'  units=units  use_header_enum=off  row_header_enum={}  col_header_enum={}  use_min_max=on  min_val=-inf  max_val=inf  use_precision=off  precision=''  gain=1  offset=0  exp=1  use_mototune_group=on  mototune_group=grp
  motohawk_calibration1 : MotoHawk_lib/Calibration & Probing Blocks/motohawk_calibration  nam=[prefix 'UprLim']  val=1  storage=Calibration  show_more=on  name_source=Use Parameter  data_type=Inherit via back propagation  read_level=1  write_level=1  ovr_cals=on  view_as=Number  enum_struct={'Disabled', 'Enabled'}  vector_style=Wide Row  use_help_units=off  help='Upper Limit Value'  units=units  use_header_enum=off  row_header_enum={}  col_header_enum={}  use_min_max=on  min_val=-inf  max_val=inf  use_precision=off  precision=''  gain=1  offset=0  exp=1  use_mototune_group=on  mototune_group=grp
  Out : Outport  OutDataType=sfix(16)  OutScaling=2^0
  wires:
  Saturation/1 -> Out/1
  motohawk_calibration/1 -> Saturation/2
  In/1 -> Saturation/1
  motohawk_calibration1/1 -> Saturation/3

== system motohawk_control_primitives_lib/Simple PD ==
  note: Simple PD Controller
  Actual : Inport  OutDataType=sfix(16)  OutScaling=2^0
  SetPt : Inport  Port=2  OutDataType=sfix(16)  OutScaling=2^0
  k_P : Inport  Port=3  OutDataType=sfix(16)  OutScaling=2^0
  k_D : Inport  Port=4  OutDataType=sfix(16)  OutScaling=2^0
  Data Type Conversion1 : DataTypeConversion  OutDataType=sfix(16)  OutScaling=2^0  SaturateOnIntegerOverflow=on  RndMeth=Zero
  Derivitive3 : motohawk_control_primitives_lib/Derivitive  samp_time=samp_time
  Model Info : simulink/Model-Wide Utilities/Model Info  InitialBlockCM=None  BlockCM=None  Frame=on  DisplayStringWithTags=|  HorizontalTextAlignment=Center  LeftAlignmentValue=0.5  SourceBlockDiagram=motohawk_control_primitives_lib  TagMaxNumber=20
      | Model Info:
      | Author: Poorman
      | %<ModifiedDate>
      | Version: %<ModelVersion>
      | MotoTron Confidential
      | and Propietary
  Product1 : Product  OutDataType=sfix(16)  OutScaling=2^0  InputSameDT=on  OutDataTypeStr=Inherit: Same as first input
  Product5 : Product  OutDataType=sfix(16)  OutScaling=2^0  InputSameDT=on  OutDataTypeStr=Inherit: Same as first input
  Sum1 : Sum  Inputs=+|+  OutDataType=sfix(16)  OutScaling=2^0  SaturateOnIntegerOverflow=on  InputSameDT=on  OutDataTypeStr=Inherit: Same as first input
  Sum2 : Sum  Inputs=-|||+  OutDataType=sfix(16)  OutScaling=2^0  SaturateOnIntegerOverflow=on  InputSameDT=on  OutDataTypeStr=Inherit: Same as first input
  Out : Outport  OutDataType=sfix(16)  OutScaling=2^0
  wires:
  Data Type Conversion1/1 -> Product5/2, Product1/1
  Actual/1 -> Sum2/1
  k_P/1 -> Product1/2
  Sum2/1 -> Data Type Conversion1/1
  SetPt/1 -> Sum2/2
  k_D/1 -> Product5/1
  Product5/1 -> Derivitive3/1
  Sum1/1 -> Out/1
  Derivitive3/1 -> Sum1/1
  Product1/1 -> Sum1/2

== system motohawk_control_primitives_lib/Simple PI ==
  note: Simple PI Controller
  Actual : Inport  OutDataType=sfix(16)  OutScaling=2^0
  SetPt : Inport  Port=2  OutDataType=sfix(16)  OutScaling=2^0
  k_P : Inport  Port=3  OutDataType=sfix(16)  OutScaling=2^0
  k_I : Inport  Port=4  OutDataType=sfix(16)  OutScaling=2^0
  Constant : Constant  OutDataType=sfix(16)  OutScaling=2^0
  Constant1 : Constant  Value=-inf  OutDataType=sfix(16)  OutScaling=2^0
  Constant2 : Constant  Value=inf  OutDataType=sfix(16)  OutScaling=2^0
  Constant3 : Constant  Value=0  OutDataType=sfix(16)  OutScaling=2^0
  Constant4 : Constant  Value=0  OutDataType=sfix(16)  OutScaling=2^0
  Data Type Conversion : DataTypeConversion  OutDataType=sfix(16)  OutScaling=2^0  SaturateOnIntegerOverflow=on  RndMeth=Zero
  Integrator : motohawk_control_primitives_lib/Integrator  samp_time=samp_time
  Model Info : simulink/Model-Wide Utilities/Model Info  InitialBlockCM=None  BlockCM=None  Frame=on  DisplayStringWithTags=|  HorizontalTextAlignment=Center  LeftAlignmentValue=0.5  SourceBlockDiagram=motohawk_control_primitives_lib  TagMaxNumber=20
      | Model Info:
      | Author: Poorman
      | %<Created>
      | %<ModifiedDate>
      | Version: %<ModelVersion>
      | MotoTron Confidential
      | and Propietary
  Product1 : Product  OutDataType=sfix(16)  OutScaling=2^0  InputSameDT=on  OutDataTypeStr=Inherit: Same as first input
  Product2 : Product  OutDataType=sfix(16)  OutScaling=2^0  InputSameDT=on  OutDataTypeStr=Inherit: Same as first input
  Product3 : Product  OutDataType=sfix(16)  OutScaling=2^0  InputSameDT=on  OutDataTypeStr=Inherit: Same as first input
  Sum : Sum  Inputs=+|+  OutDataType=sfix(16)  OutScaling=2^0  SaturateOnIntegerOverflow=on  InputSameDT=on  OutDataTypeStr=Inherit: Same as first input
  Sum2 : Sum  Inputs=-|+  OutDataType=sfix(16)  OutScaling=2^0  SaturateOnIntegerOverflow=on  InputSameDT=on  OutDataTypeStr=Inherit: Same as first input
  Out : Outport  OutDataType=sfix(16)  OutScaling=2^0
  wires:
  Constant2/1 -> Integrator/5
  Constant1/1 -> Integrator/4
  Data Type Conversion/1 -> Product3/1
  Constant/1 -> Product3/2
  Constant4/1 -> Integrator/2
  SetPt/1 -> Sum2/2
  Actual/1 -> Sum2/1
  k_P/1 -> Product2/1
  k_I/1 -> Product1/2
  Product1/1 -> Integrator/1
  Product2/1 -> Sum/1
  Integrator/1 -> Sum/2
  Sum/1 -> Out/1
  Constant3/1 -> Integrator/3
  Product3/1 -> Product2/2, Product1/1
  Sum2/1 -> Data Type Conversion/1

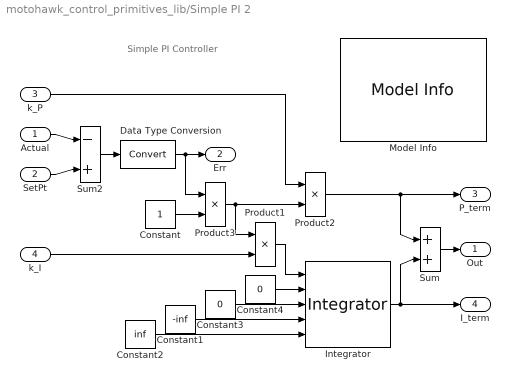
== system motohawk_control_primitives_lib/Simple PI 2 ==
  note: Simple PI Controller
  Actual : Inport  OutDataType=sfix(16)  OutScaling=2^0
  SetPt : Inport  Port=2  OutDataType=sfix(16)  OutScaling=2^0
  k_P : Inport  Port=3  OutDataType=sfix(16)  OutScaling=2^0
  k_I : Inport  Port=4  OutDataType=sfix(16)  OutScaling=2^0
  Constant : Constant  OutDataType=sfix(16)  OutScaling=2^0
  Constant1 : Constant  Value=-inf  OutDataType=sfix(16)  OutScaling=2^0
  Constant2 : Constant  Value=inf  OutDataType=sfix(16)  OutScaling=2^0
  Constant3 : Constant  Value=0  OutDataType=sfix(16)  OutScaling=2^0
  Constant4 : Constant  Value=0  OutDataType=sfix(16)  OutScaling=2^0
  Data Type Conversion : DataTypeConversion  OutDataType=sfix(16)  OutScaling=2^0  SaturateOnIntegerOverflow=on  RndMeth=Zero
  Integrator : motohawk_control_primitives_lib/Integrator  samp_time=samp_time
  Model Info : simulink/Model-Wide Utilities/Model Info  InitialBlockCM=None  BlockCM=None  Frame=on  DisplayStringWithTags=|  HorizontalTextAlignment=Center  LeftAlignmentValue=0.5  SourceBlockDiagram=motohawk_control_primitives_lib  TagMaxNumber=20
      | Model Info:
      | Author: Poorman
      | %<Created>
      | %<ModifiedDate>
      | Version: %<ModelVersion>
      | MotoTron Confidential
      | and Propietary
  Product1 : Product  OutDataType=sfix(16)  OutScaling=2^0  InputSameDT=on  OutDataTypeStr=Inherit: Same as first input
  Product2 : Product  OutDataType=sfix(16)  OutScaling=2^0  InputSameDT=on  OutDataTypeStr=Inherit: Same as first input
  Product3 : Product  OutDataType=sfix(16)  OutScaling=2^0  InputSameDT=on  OutDataTypeStr=Inherit: Same as first input
  Sum : Sum  Inputs=+|+  OutDataType=sfix(16)  OutScaling=2^0  SaturateOnIntegerOverflow=on  InputSameDT=on  OutDataTypeStr=Inherit: Same as first input
  Sum2 : Sum  Inputs=-|+  OutDataType=sfix(16)  OutScaling=2^0  SaturateOnIntegerOverflow=on  InputSameDT=on  OutDataTypeStr=Inherit: Same as first input
  Out : Outport  OutDataType=sfix(16)  OutScaling=2^0
  Err : Outport  Port=2  OutDataType=sfix(16)  OutScaling=2^0
  P_term : Outport  Port=3  OutDataType=sfix(16)  OutScaling=2^0
  I_term : Outport  Port=4  OutDataType=sfix(16)  OutScaling=2^0
  wires:
  Sum2/1 -> Data Type Conversion/1
  Product3/1 -> Product1/1, Product2/2
  Constant3/1 -> Integrator/3
  Sum/1 -> Out/1
  Integrator/1 -> Sum/2, I_term/1
  Product2/1 -> Sum/1, P_term/1
  Product1/1 -> Integrator/1
  k_I/1 -> Product1/2
  k_P/1 -> Product2/1
  Actual/1 -> Sum2/1
  SetPt/1 -> Sum2/2
  Constant4/1 -> Integrator/2
  Constant/1 -> Product3/2
  Data Type Conversion/1 -> Product3/1, Err/1
  Constant1/1 -> Integrator/4
  Constant2/1 -> Integrator/5

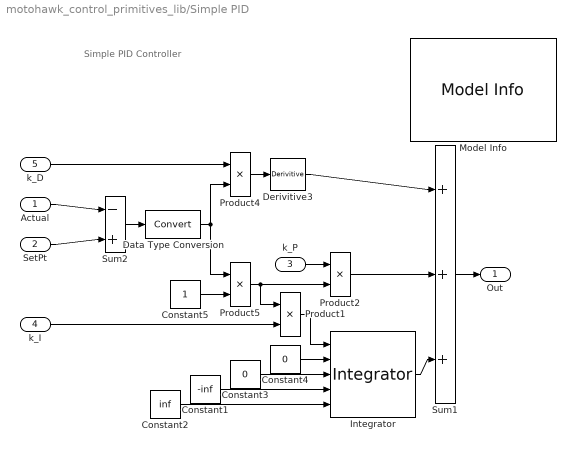
== system motohawk_control_primitives_lib/Simple PID ==
  note: Simple PID Controller
  Actual : Inport  OutDataType=sfix(16)  OutScaling=2^0
  SetPt : Inport  Port=2  OutDataType=sfix(16)  OutScaling=2^0
  k_P : Inport  Port=3  OutDataType=sfix(16)  OutScaling=2^0
  k_I : Inport  Port=4  OutDataType=sfix(16)  OutScaling=2^0
  k_D : Inport  Port=5  OutDataType=sfix(16)  OutScaling=2^0
  Constant1 : Constant  Value=-inf  OutDataType=sfix(16)  OutScaling=2^0
  Constant2 : Constant  Value=inf  OutDataType=sfix(16)  OutScaling=2^0
  Constant3 : Constant  Value=0  OutDataType=sfix(16)  OutScaling=2^0
  Constant4 : Constant  Value=0  OutDataType=sfix(16)  OutScaling=2^0
  Constant5 : Constant  OutDataType=sfix(16)  OutScaling=2^0
  Data Type Conversion : DataTypeConversion  OutDataType=sfix(16)  OutScaling=2^0  SaturateOnIntegerOverflow=on  RndMeth=Zero
  Derivitive3 : motohawk_control_primitives_lib/Derivitive  samp_time=samp_time
  Integrator : motohawk_control_primitives_lib/Integrator  samp_time=samp_time
  Model Info : simulink/Model-Wide Utilities/Model Info  InitialBlockCM=None  BlockCM=None  Frame=on  DisplayStringWithTags=|  HorizontalTextAlignment=Center  LeftAlignmentValue=0.5  SourceBlockDiagram=motohawk_control_primitives_lib  TagMaxNumber=20
      | Model Info:
      | Author: Suhre, Poorman
      | %<Created>
      | %<ModifiedDate>
      | Version: %<ModelVersion>
      | MotoTron Confidential
      | and Propietary
  Product{1..2,4..5} (4 alike) : Product  OutDataType=sfix(16)  OutScaling=2^0  InputSameDT=on  OutDataTypeStr=Inherit: Same as first input
  Sum1 : Sum  Inputs=+|+|+  OutDataType=sfix(16)  OutScaling=2^0  SaturateOnIntegerOverflow=on  InputSameDT=on  OutDataTypeStr=Inherit: Same as first input
  Sum2 : Sum  Inputs=-|+  OutDataType=sfix(16)  OutScaling=2^0  SaturateOnIntegerOverflow=on  InputSameDT=on  OutDataTypeStr=Inherit: Same as first input
  Out : Outport  OutDataType=sfix(16)  OutScaling=2^0
  wires:
  Data Type Conversion/1 -> Product5/1, Product4/2
  Constant5/1 -> Product5/2
  Actual/1 -> Sum2/1
  k_P/1 -> Product2/1
  k_I/1 -> Product1/2
  Product1/1 -> Integrator/1
  Product2/1 -> Sum1/2
  Integrator/1 -> Sum1/3
  Sum1/1 -> Out/1
  Product5/1 -> Product2/2, Product1/1
  Sum2/1 -> Data Type Conversion/1
  SetPt/1 -> Sum2/2
  k_D/1 -> Product4/1
  Product4/1 -> Derivitive3/1
  Derivitive3/1 -> Sum1/1
  Constant2/1 -> Integrator/5
  Constant1/1 -> Integrator/4
  Constant3/1 -> Integrator/3
  Constant4/1 -> Integrator/2
